simulink library "Autonomous_lib"  (R2023b)
settings: Solver=VariableStepAuto  StartTime=0.0  StopTime=10.0  RelTol=1e-3
undefined symbols (not defined in the file): Autonomous_Desired_X, Autonomous_Desired_Y, Spline_Num_Poses_auto, Spline_Ref_Poses_auto, t_sample
settings Model: Creator=FIRSTMentor  LastModifiedBy=ander

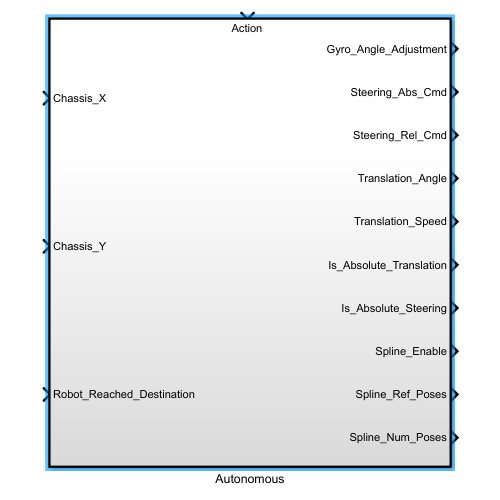
[thumbnail: Simulink's stored preview of the top-level diagram]
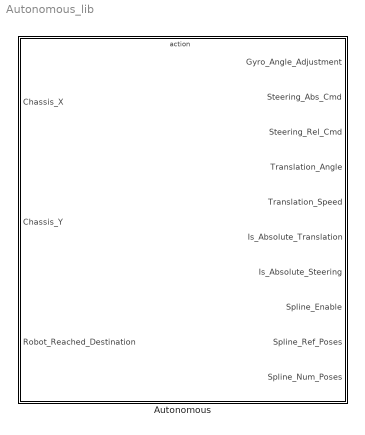
== system Autonomous_lib ==
  Autonomous : Subsystem  TreatAsAtomicUnit=on

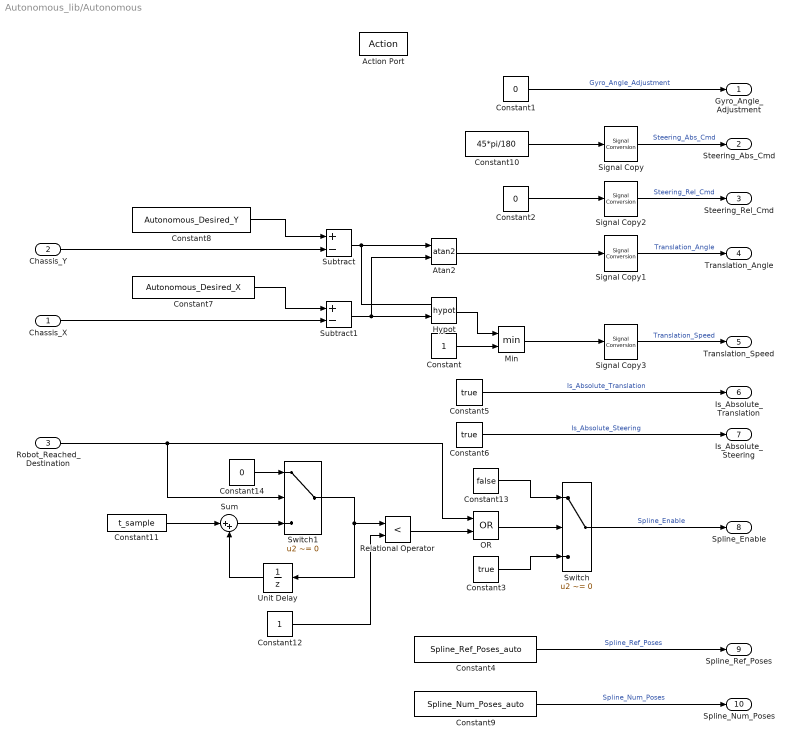
== system Autonomous_lib/Autonomous ==
  Chassis_X : Inport
  Chassis_Y : Inport  Port=2
  Robot_Reached_Destination : Inport  Port=3
  Action Port : ActionPort  InitializeStates=reset
  Atan2 : Trigonometry  Operator=atan2
  Constant : Constant
  Constant1 : Constant  Value=0
  Constant10 : Constant  Value=45*pi/180
  Constant11 : Constant  Value=t_sample
  Constant12 : Constant
  Constant13 : Constant  Value=false  OutDataTypeStr=boolean
  Constant14 : Constant  Value=0
  Constant2 : Constant  Value=0
  Constant3 : Constant  Value=true  OutDataTypeStr=boolean
  Constant4 : Constant  Value=Spline_Ref_Poses_auto
  Constant5 : Constant  Value=true
  Constant6 : Constant  Value=true
  Constant7 : Constant  Value=Autonomous_Desired_X
  Constant8 : Constant  Value=Autonomous_Desired_Y
  Constant9 : Constant  Value=Spline_Num_Poses_auto  OutDataTypeStr=double
  Hypot : Math  Operator=hypot
  Min : MinMax  Inputs=2
  OR : Logic  Operator=OR  AllPortsSameDT=off  OutDataTypeStr=boolean
  Relational Operator : RelationalOperator  Operator=<  OutDataTypeStr=boolean  RndMeth=Simplest  InputSameDT=off
  Signal Copy{,1..3} (4 alike) : SignalConversion  OverrideOpt=off
  Subtract : Sum  Inputs=+-
  Subtract1 : Sum  Inputs=+-
  Sum : Sum  Inputs=|++
  Switch : Switch  Criteria=u2 ~= 0  SaturateOnIntegerOverflow=off  InputSameDT=off
  Switch1 : Switch  Criteria=u2 ~= 0  SaturateOnIntegerOverflow=off  InputSameDT=off
  Unit Delay : UnitDelay  SampleTime=-1  HasFrameUpgradeWarning=on
  Gyro_Angle_Adjustment : Outport
  Steering_Abs_Cmd : Outport  Port=2
  Steering_Rel_Cmd : Outport  Port=3
  Translation_Angle : Outport  Port=4
  Translation_Speed : Outport  Port=5
  Is_Absolute_Translation : Outport  Port=6
  Is_Absolute_Steering : Outport  Port=7
  Spline_Enable : Outport  Port=8
  Spline_Ref_Poses : Outport  Port=9
  Spline_Num_Poses : Outport  Port=10
  wires:
  Constant6/1 -> Is_Absolute_Steering/1  "Is_Absolute_Steering"
  Hypot/1 -> Min/1
  Constant8/1 -> Subtract/1
  Chassis_Y/1 -> Subtract/2
  Constant7/1 -> Subtract1/1
  Signal Copy/1 -> Steering_Abs_Cmd/1  "Steering_Abs_Cmd"
  Chassis_X/1 -> Subtract1/2
  Constant5/1 -> Is_Absolute_Translation/1  "Is_Absolute_Translation"
  Signal Copy1/1 -> Translation_Angle/1  "Translation_Angle"
  Constant2/1 -> Signal Copy2/1
  Subtract/1 -> Hypot/1, Atan2/1
  Subtract1/1 -> Hypot/2, Atan2/2
  Constant10/1 -> Signal Copy/1
  Constant/1 -> Min/2
  Constant1/1 -> Gyro_Angle_Adjustment/1  "Gyro_Angle_Adjustment"
  Constant4/1 -> Spline_Ref_Poses/1  "Spline_Ref_Poses"
  Constant9/1 -> Spline_Num_Poses/1  "Spline_Num_Poses"
  Signal Copy2/1 -> Steering_Rel_Cmd/1  "Steering_Rel_Cmd"
  Signal Copy3/1 -> Translation_Speed/1  "Translation_Speed"
  Min/1 -> Signal Copy3/1
  Atan2/1 -> Signal Copy1/1
  Constant11/1 -> Sum/1
  Unit Delay/1 -> Sum/2
  Constant12/1 -> Relational Operator/2
  Switch/1 -> Spline_Enable/1  "Spline_Enable"
  Relational Operator/1 -> OR/2
  OR/1 -> Switch/2
  Robot_Reached_Destination/1 -> OR/1, Switch1/2
  Constant13/1 -> Switch/1
  Constant3/1 -> Switch/3
  Sum/1 -> Switch1/3
  Switch1/1 -> Relational Operator/1, Unit Delay/1
  Constant14/1 -> Switch1/1
